simulink model "prelim_FFT"  (R2013a)
settings: Solver=ode45  StartTime=0.0  StopTime=10000  RelTol=1e-3
PostLoadFcn:
  | bps_model_init(gcs);
undefined symbols (not defined in the file or in its folder): xlipgetpartsetting
libraries: xbsIndex_r4 x75, xps_library x22, mbee4_library x4
(part 1 of 3)
settings Model: Creator=BEEcube  LastModifiedBy=rijesh
settings DataIOCC: SignalLoggingSaveFormat=ModelDataLogs
settings OptimizationCC: InlineParams=on  ExpressionDepthLimit=2147483647
settings DebuggingCC: FcnCallInpInsideContextMsg=UseLocalSettings
settings GRTTargetCC: CombineOutputUpdateFcns=off  GRTInterface=on

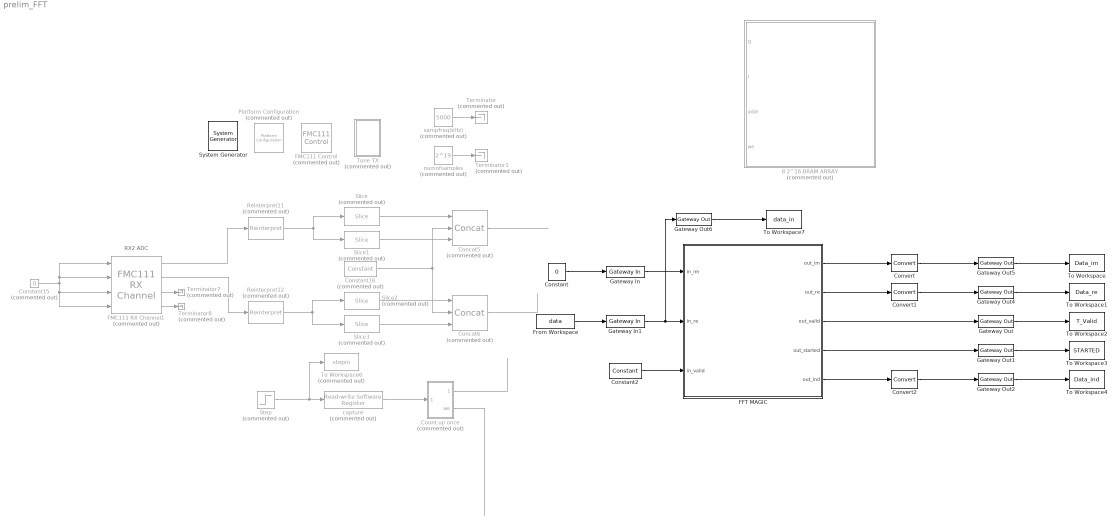
== system prelim_FFT ==
  note: RX2 ADC
  " Platform Configuration " : mbee4_library/ Platform Configuration   Tag=xps:xsg,ver:4.5  Commented=on  xsg_ver=14.7  hw_sys=mBEE4  fpga_type=xc6vsx475t  fpga_device='xc6vsx475t-2ff1759'  bp_override=off  bp_choice='mBEE4'  bp_option=base  clk_src=fmc_clk1_fx: User defined clock based on FMC_HPC_CLK1  clk_rate=250000000  ref_clk_rate=250000000  enable_half_rate=off  sample_period=1  update=off
  " System Generator" : xbsIndex_r4/ System Generator  Tag=genX  xilinxfamily=virtex6  part=xc6vsx475t  speed=-2  package=ff1759  synthesis_tool=XST  clock_wrapper=Clock Enables  directory=./radarDFT/sysgen  proj_type=Project Navigator  Synth_file=XST Defaults  Impl_file=ISE Defaults  testbench=off  simulink_period=1  sysclk_period=4  dcm_input_clock_period=10  incr_netlist=off  trim_vbits=Everywhere in SubSystem  dbl_ovrd=According to Block Masks  core_generation=According to Block Masks  run_coregen=off  deprecated_control=off  eval_field=0  block_type=sysgen
  8 2^16 BRAM ARRAY : Subsystem  Commented=on
  Concat5 : xbsIndex_r4/Concat  Commented=on  num_inputs=3  dbl_ovrd=off  block_type=concat
  Concat6 : xbsIndex_r4/Concat  Commented=on  num_inputs=3  dbl_ovrd=off  block_type=concat
  Constant : Constant  Value=0
  Constant15 : Constant  Commented=on  Value=0  SampleTime=1
  Constant16 : xbsIndex_r4/Constant  Commented=on  const=0  gui_display_data_type=Fixed-point  arith_type=Unsigned  n_bits=18  bin_pt=0  preci_type=Single  exp_width=8  frac_width=24  explicit_period=off  period=1  equ=P=C  opselect=C  inp2=PCIN>>17  opr=+  inp1=P  carry=CIN  dbl_ovrd=off  block_type=constant
  Constant2 : xbsIndex_r4/Constant  const=1  gui_display_data_type=Boolean  arith_type=Boolean  n_bits=16  bin_pt=0  preci_type=Single  exp_width=8  frac_width=24  explicit_period=off  period=1  equ=P=C  opselect=C  inp2=PCIN>>17  opr=+  inp1=P  carry=CIN  dbl_ovrd=off  block_type=constant
  Convert : xbsIndex_r4/Convert  gui_display_data_type=Fixed-point  arith_type="Signed  (2's comp)"  n_bits=16  bin_pt=15  float_type=Double  exp_bits=8  fraction_bits=24  quantization=Truncate  overflow=Wrap  en=off  latency=0  dbl_ovrd=off  pipeline=off  block_type=convert
  Convert1 : xbsIndex_r4/Convert  gui_display_data_type=Fixed-point  arith_type="Signed  (2's comp)"  n_bits=16  bin_pt=15  float_type=Double  exp_bits=8  fraction_bits=24  quantization=Truncate  overflow=Wrap  en=off  latency=0  dbl_ovrd=off  pipeline=off  block_type=convert
  Convert2 : xbsIndex_r4/Convert  gui_display_data_type=Fixed-point  arith_type=Unsigned  n_bits=8  bin_pt=0  float_type=Double  exp_bits=8  fraction_bits=24  quantization=Truncate  overflow=Wrap  en=off  latency=0  dbl_ovrd=off  pipeline=off  block_type=convert
  Count up once : Subsystem  Commented=on
  FFT MAGIC : Subsystem
  FMC111 Control : mbee4_library/FMC111 Control  Tag=xps:fmc111_ctrl  Commented=on  board_type=FMC111  sample_period=1  update=off
  FMC111 RX Channel1 : mbee4_library/FMC111 RX Channel  Tag=xps:fmc111_rx  Commented=on  channel_number=1  arith_type=Signed  bitwidth=14  bin_pt=0  sample_period=1  update=off
  From Workspace : FromWorkspace  VariableName=data  SampleTime=0
  Gateway In : xbsIndex_r4/Gateway In  gui_display_data_type=Fixed-point  arith_type="Signed  (2's comp)"  n_bits=16  bin_pt=15  preci_type=Single  exp_width=8  frac_width=24  quantization="Round  (unbiased: +/- Inf)"  overflow=Saturate  period=1  dbl_ovrd=off  timing_constraint=None  locs_specified=off  LOCs={}  UseAsADC=off  ADCChannel='1'  inherit_from_input=off  hdl_port=on  block_type=gatewayin
  Gateway In1 : xbsIndex_r4/Gateway In  gui_display_data_type=Fixed-point  arith_type="Signed  (2's comp)"  n_bits=16  bin_pt=15  preci_type=Single  exp_width=8  frac_width=24  quantization="Round  (unbiased: +/- Inf)"  overflow=Saturate  period=1  dbl_ovrd=off  timing_constraint=None  locs_specified=off  LOCs={}  UseAsADC=off  ADCChannel='1'  inherit_from_input=off  hdl_port=on  block_type=gatewayin
  Gateway Out{,1..2,4..6} (6 alike) : xbsIndex_r4/Gateway Out  inherit_from_input=off  hdl_port=on  timing_constraint=None  locs_specified=off  LOCs={}  UseAsDAC=off  DACChannel='1'  block_type=gatewayout
  Reinterpret11 : xbsIndex_r4/Reinterpret  Commented=on  force_arith_type=on  arith_type=Unsigned  force_bin_pt=off  bin_pt=0  block_type=reinterpret
  Reinterpret12 : xbsIndex_r4/Reinterpret  Commented=on  force_arith_type=on  arith_type=Unsigned  force_bin_pt=off  bin_pt=0  block_type=reinterpret
  Slice : xbsIndex_r4/Slice  Commented=on  nbits=1  boolean_output=off  mode=Upper Bit Location + Width  bit1=0  base1=MSB of Input  bit0=0  base0=LSB of Input  dbl_ovrd=off  block_type=slice
  Slice1 : xbsIndex_r4/Slice  Commented=on  nbits=13  boolean_output=off  mode=Lower Bit Location + Width  bit1=0  base1=MSB of Input  bit0=0  base0=LSB of Input  dbl_ovrd=off  block_type=slice
  Slice2 : xbsIndex_r4/Slice  Commented=on  nbits=1  boolean_output=off  mode=Upper Bit Location + Width  bit1=0  base1=MSB of Input  bit0=0  base0=LSB of Input  dbl_ovrd=off  block_type=slice
  Slice3 : xbsIndex_r4/Slice  Commented=on  nbits=13  boolean_output=off  mode=Lower Bit Location + Width  bit1=0  base1=MSB of Input  bit0=0  base0=LSB of Input  dbl_ovrd=off  block_type=slice
  Step : Step  Commented=on  SampleTime=1
  Terminator{,1,7..8} (4 alike) : Terminator  Commented=on
  To Workspace : ToWorkspace  VariableName=Data_im  SampleTime=-1  SaveFormat=Timeseries
  To Workspace1 : ToWorkspace  VariableName=Data_re  SampleTime=-1  SaveFormat=Timeseries
  To Workspace2 : ToWorkspace  VariableName=T_Valid  SampleTime=-1  SaveFormat=Timeseries
  To Workspace3 : ToWorkspace  VariableName=STARTED  SampleTime=-1  SaveFormat=Timeseries
  To Workspace4 : ToWorkspace  VariableName=Data_ind  SampleTime=-1  SaveFormat=Timeseries
  To Workspace6 : ToWorkspace  Commented=on  VariableName=stepin  SampleTime=-1
  To Workspace7 : ToWorkspace  VariableName=data_in  SampleTime=-1  SaveFormat=Timeseries
  Tone TX : Subsystem  Commented=on  VariantControl=Variant1
  capture : xps_library/Read-write Software Register  Tag=xps:sw_reg  Commented=on  io_dir=From Processor  use_strobe=off  arith_type=Unsigned  bitwidth=32  bin_pt=0  sample_period=1  update=off
  numofsamples : Constant  Commented=on  Value=2^19
  sampfreq(kHz) : Constant  Commented=on  Value=5000
  wires:
  Step/1 -> capture/1, To Workspace6/1
  Constant15/1 -> FMC111 RX Channel1/1, FMC111 RX Channel1/2, FMC111 RX Channel1/4, FMC111 RX Channel1/3
  FMC111 RX Channel1/3 -> Terminator7/1
  FMC111 RX Channel1/4 -> Terminator8/1
  FMC111 RX Channel1/1 -> Reinterpret11/1
  FMC111 RX Channel1/2 -> Reinterpret12/1
  Reinterpret11/1 -> Slice1/1, Slice/1
  Reinterpret12/1 -> Slice2/1, Slice3/1
  Constant16/1 -> Concat5/2, Concat6/2
  Concat5/1 -> ?
  Concat6/1 -> ?
  sampfreq(kHz)/1 -> Terminator/1
  numofsamples/1 -> Terminator1/1
  capture/1 -> Count up once/1(start)
  Count up once/1(addr) -> ?
  Count up once/2(we) -> ?
  Slice/1 -> Concat5/1
  Slice1/1 -> Concat5/3
  Slice3/1 -> Concat6/3
  Slice2/1 -> Concat6/1
  Constant2/1 -> FFT MAGIC/3(in_valid)
  Gateway In/1 -> FFT MAGIC/1(in_im)
  Gateway In1/1 -> Gateway Out6/1, FFT MAGIC/2(in_re)
  FFT MAGIC/5(out_ind) -> Convert2/1
  FFT MAGIC/4(out_started) -> Gateway Out1/1
  FFT MAGIC/3(out_valid) -> Gateway Out/1
  FFT MAGIC/1(out_im) -> Convert/1
  FFT MAGIC/2(out_re) -> Convert1/1
  From Workspace/1 -> Gateway In1/1
  Constant/1 -> Gateway In/1
  Gateway Out5/1 -> To Workspace/1
  Gateway Out4/1 -> To Workspace1/1
  Gateway Out/1 -> To Workspace2/1
  Gateway Out1/1 -> To Workspace3/1
  Gateway Out2/1 -> To Workspace4/1
  Convert1/1 -> Gateway Out4/1
  Convert/1 -> Gateway Out5/1
  Gateway Out6/1 -> To Workspace7/1
  Convert2/1 -> Gateway Out2/1
